simulink model "Diode_Bridge_PSFB"  (R2022a)
settings: Solver=ode4  StartTime=0.0  StopTime=0.1  FixedStep=1e-9  RelTol=1e-3
undefined symbols (not defined in the file): C_PSFB, Gci_inf, Gcv_inf, H_PSFB, L_PSFB, Rsense_PSFB, Vin_PSFB, wLi_PSFB, wLv_PSFB
libraries: spsDiodeLib x4, spsMosfetLib x4, spsSeriesRLCBranchLib x3, spsCurrentMeasurementLib x1, spsLinearTransformerLib x1, spsDCVoltageSourceLib x1, spsVoltageMeasurementLib x1, spspowerguiLib x1
settings Model: Creator=Aditya Bhalotia  LastModifiedBy=Aditya Bhalotia

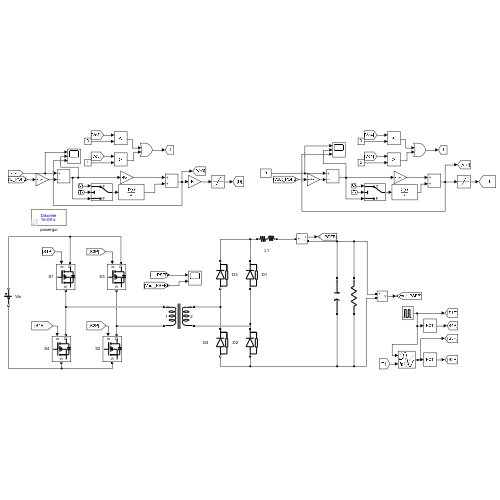
[thumbnail: Simulink's stored preview of the top-level diagram]
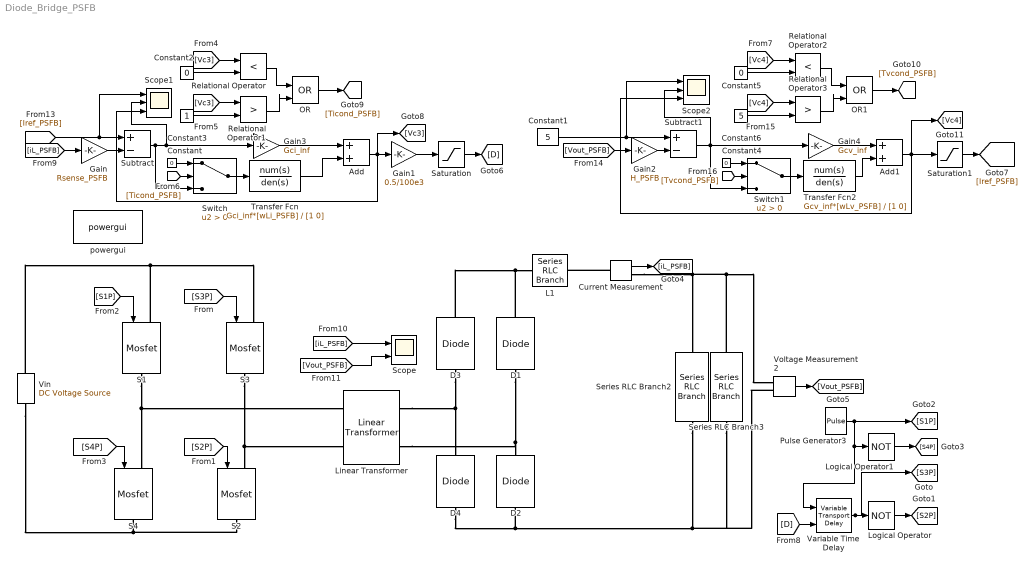
== system Diode_Bridge_PSFB ==
  Add : Sum
  Add1 : Sum
  Constant{,2,4..5} (4 alike) : Constant  Value=0
  Constant1 : Constant  Value=5
  Constant3 : Constant
  Constant6 : Constant  Value=5
  Current Measurement : spsCurrentMeasurementLib/Current Measurement  PhasorSimulation=off  OutputType=Complex  PSBequivalent=0
  D{1..4} (4 alike) : spsDiodeLib/Diode  Ron=0.001  Lon=0  Vf=1  IC=0  UseSnubber=0  Rs=500e6  Cs=1e-15  Measurements=off
  Gain : Gain  Gain=Rsense_PSFB
  Gain1 : Gain  Gain=0.5/100e3
  Gain2 : Gain  Gain=H_PSFB
  Gain3 : Gain  Gain=Gci_inf
  Gain4 : Gain  Gain=Gcv_inf
  L1 : spsSeriesRLCBranchLib/Series RLC Branch  LConnTagsString=__new0  RConnTagsString=__new0  BranchType=RL  Resistance=0  Inductance=L_PSFB  SetiL0=off  InitialCurrent=0  Capacitance=1e-6  Setx0=off  InitialVoltage=0  Measurements=Branch current
  Linear Transformer : spsLinearTransformerLib/Linear Transformer  UNITS=SI  NominalPower=[50e2 100e3]  winding1=[400 0.01 0]  winding2=[400 0.01 0]  ThreeWindings=off  winding3=[3.15e+05 0.7938 0.084225]  RmLm=[1.0804e5 28e-3]  Measurements=None  DataType=on
  Logical Operator : Logic  Operator=NOT  AllPortsSameDT=off  OutDataTypeStr=boolean
  Logical Operator1 : Logic  Operator=NOT  AllPortsSameDT=off  OutDataTypeStr=boolean
  OR : Logic  Operator=OR  IconShape=distinctive  AllPortsSameDT=off  OutDataTypeStr=boolean
  OR1 : Logic  Operator=OR  IconShape=distinctive  AllPortsSameDT=off  OutDataTypeStr=boolean
  Pulse Generator3 : DiscretePulseGenerator  PulseType=Time based  Amplitude=15  Period=10e-6  PulseWidth=50
  Relational Operator : RelationalOperator  Operator=<  OutDataTypeStr=boolean  RndMeth=Simplest  InputSameDT=off
  Relational Operator1 : RelationalOperator  Operator=>  OutDataTypeStr=boolean  RndMeth=Simplest  InputSameDT=off
  Relational Operator2 : RelationalOperator  Operator=<  OutDataTypeStr=boolean  RndMeth=Simplest  InputSameDT=off
  Relational Operator3 : RelationalOperator  Operator=>  OutDataTypeStr=boolean  RndMeth=Simplest  InputSameDT=off
  S{1..4} (4 alike) : spsMosfetLib/Mosfet  Ron=0.001  Lon=0  Rd=0.01  Vfd=0  IC=0  Rs=1e5  Cs=inf  Measurements=off
  Saturation : Saturate  UpperLimit=5e-6  LowerLimit=0
  Saturation1 : Saturate  UpperLimit=5  LowerLimit=0
  Scope : Scope  NumInputPorts=2
  Scope1 : Scope  NumInputPorts=3
  Scope2 : Scope  NumInputPorts=3
  Series RLC Branch2 : spsSeriesRLCBranchLib/Series RLC Branch  LConnTagsString=__new0  RConnTagsString=__new0  BranchType=C  Resistance=1  Inductance=1e-3  SetiL0=off  InitialCurrent=0  Capacitance=C_PSFB  Setx0=off  InitialVoltage=0  Measurements=None
  Series RLC Branch3 : spsSeriesRLCBranchLib/Series RLC Branch  LConnTagsString=__new0  RConnTagsString=__new0  BranchType=R  Resistance=313.6  Inductance=1e-3  SetiL0=off  InitialCurrent=0  Capacitance=1e-6  Setx0=off  InitialVoltage=0  Measurements=None
  Subtract : Sum  Inputs=+-
  Subtract1 : Sum  Inputs=+-
  Switch : Switch  Criteria=u2 > Threshold  SaturateOnIntegerOverflow=off  InputSameDT=off
  Switch1 : Switch  Criteria=u2 > Threshold  SaturateOnIntegerOverflow=off  InputSameDT=off
  Transfer Fcn : TransferFcn  Numerator=Gci_inf*[wLi_PSFB]  Denominator=[1 0]
  Transfer Fcn2 : TransferFcn  Numerator=Gcv_inf*[wLv_PSFB]  Denominator=[1 0]
  Variable Time Delay : VariableTransportDelay  MaximumDelay=5.1e-6
  Vin : spsDCVoltageSourceLib/DC Voltage Source  Amplitude=Vin_PSFB  Measurements=None
  Voltage Measurement2 : spsVoltageMeasurementLib/Voltage Measurement  PhasorSimulation=off  OutputType=Complex  PSBequivalent=0
  powergui : spspowerguiLib/powergui  Priority=1  SimulationMode=Discrete  SampleTime=1e-9  frequency=60  Iterations=50  frequencyindice=0  Pbase=100e6  ErrMax=1e-4  UnitsV=kV  UnitsW=MW  buscounter=0  FunctionMessages=off  echomessages=off  EnableUseOfTLC=off  CurrentSourceSwitches=off  DisableSnubberDevices=off  DisableRonSwitches=off  DisableVfSwitches=off  DisplayEquations=off  AutomaticDiscreteSolvers=off  SolverType=Tustin/Backward Euler (TBE)  Interpol=off  ExternalGateDelay=off  methode=off  Ts=100  x0status=blocks  SPID=on  SwTol=0  HookPort=off  NonlinearTolerance=1e-4  nMaxIteration=100  ContinueOnMaxIteration=off  RestoreLinks=warning  ResistiveCurrentMeasurement=off  Frange=[0:2:500]  Ylog=off  Xlog=on  ShowGrid=off  save=off  variable=ZData  structure=0  ZoomFFT=off  StartTime=0.0  cycles=1  DisplayStyle=1  fundamental=60  FreqAxis=off  MaxFrequency=1000  frequencyindicesteady=1  RmsSteady=1  display=off
  wires:
  [S1P] -> S1/1
  [S4P] -> S4/1
  [S3P] -> S3/1
  [S2P] -> S2/1
  Variable Time Delay/1 -> [S3P], Logical Operator/1
  Logical Operator/1 -> [S2P]
  Logical Operator1/1 -> [S4P]
  Pulse Generator3/1 -> Variable Time Delay/1, Logical Operator1/1, [S1P]
  Current Measurement/1 -> [iL_PSFB]
  Voltage Measurement2/1 -> [Vout_PSFB]
  [D] -> Variable Time Delay/2
  [iL_PSFB] -> Gain/1
  [Iref_PSFB] -> Scope1/1, Subtract/1
  Gain/1 -> Subtract/2
  Subtract/1 -> Switch/3, Scope1/2, Gain3/1
  Gain1/1 -> Saturation/1
  [iL_PSFB] -> Scope/1
  [Vout_PSFB] -> Scope/2
  Saturation/1 -> [D]
  Gain2/1 -> Subtract1/2
  Saturation1/1 -> [Iref_PSFB]
  [Vout_PSFB] -> Gain2/1
  Constant1/1 -> Scope2/1, Subtract1/1
  Switch/1 -> Transfer Fcn/1
  Gain3/1 -> Add/1
  Transfer Fcn/1 -> Add/2
  Constant/1 -> Switch/1
  Add/1 -> [Vc3], Scope1/3, Gain1/1
  [Vc3] -> Relational Operator/1
  Constant2/1 -> Relational Operator/2
  [Vc3] -> Relational Operator1/1
  Constant3/1 -> Relational Operator1/2
  Relational Operator/1 -> OR/1
  Relational Operator1/1 -> OR/2
  OR/1 -> [Ticond_PSFB]
  [Ticond_PSFB] -> Switch/2
  [Tvcond_PSFB] -> Switch1/2
  Relational Operator3/1 -> OR1/2
  Constant6/1 -> Relational Operator3/2
  [Vc4] -> Relational Operator3/1
  OR1/1 -> [Tvcond_PSFB]
  [Vc4] -> Relational Operator2/1
  Relational Operator2/1 -> OR1/1
  Switch1/1 -> Transfer Fcn2/1
  Constant5/1 -> Relational Operator2/2
  Constant4/1 -> Switch1/1
  Subtract1/1 -> Scope2/2, Switch1/3, Gain4/1
  Transfer Fcn2/1 -> Add1/2
  Gain4/1 -> Add1/1
  Add1/1 -> [Vc4], Scope2/3, Saturation1/1
  connections:
  S3/RConn1 -- Linear Transformer/LConn2 -- S2/LConn1
  D4/LConn1 -- Voltage Measurement2/LConn2 -- Series RLC Branch3/RConn1 -- Series RLC Branch2/RConn1 -- D2/LConn1
  D1/RConn1 -- D3/RConn1 -- L1/LConn1
  Series RLC Branch3/LConn1 -- Current Measurement/RConn1 -- Series RLC Branch2/LConn1 -- Voltage Measurement2/LConn1
  Vin/LConn1 -- S2/RConn1 -- S4/RConn1
  Vin/RConn1 -- S1/LConn1 -- S3/LConn1
  Current Measurement/LConn1 -- L1/RConn1
  S1/RConn1 -- Linear Transformer/LConn1 -- S4/LConn1
  D1/LConn1 -- Linear Transformer/RConn2 -- D2/RConn1
  D3/LConn1 -- D4/RConn1 -- Linear Transformer/RConn1
